simulink model "VAB_non_linear_Discrete"  (R2019b)
settings: Solver=FixedStepAuto  StartTime=0.0  StopTime=t_end  FixedStep=Ts  RelTol=1e-3
undefined symbols (not defined in the file or in its folder): Discrete, m_c_simulazione, phi_iniziale, phi_p_iniziale, phi_p_setpoint, phi_secondo, sensitivity_encoder, sensitivity_giroscopio, theta_iniziale, theta_p_iniziale, theta_secondo, Time, Ts
libraries: simulink x2, ctrlSharedLib x2
settings Model: Creator=miche  LastModifiedBy=AndreaCalegari

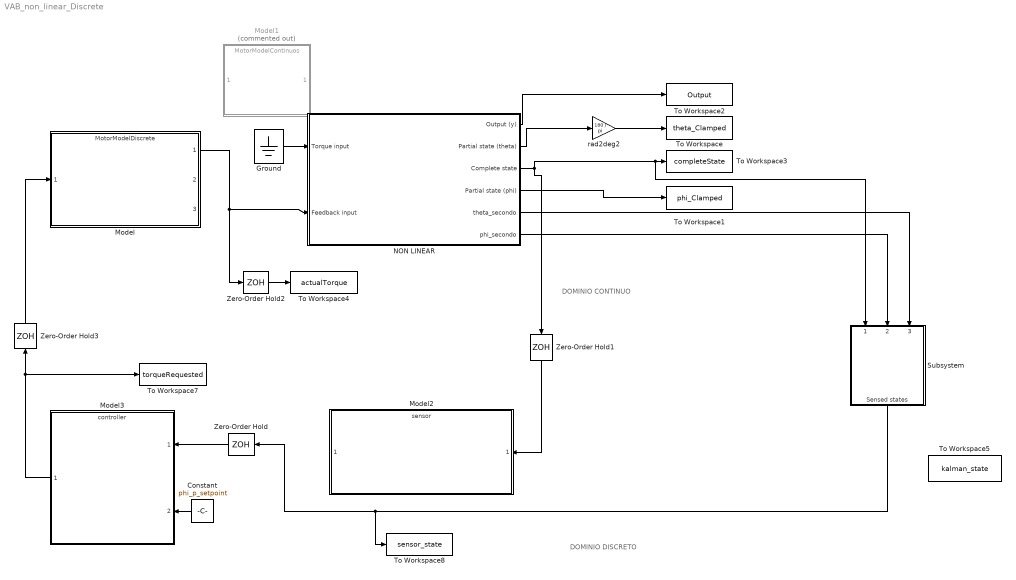
== system VAB_non_linear_Discrete ==
  note: DOMINIO DISCRETO
  note: DOMINIO CONTINUO
  Constant : Constant  Value=phi_p_setpoint
  Ground : Ground
  Model : ModelReference  ModelNameDialog=MotorModelDiscrete.slx  SimulationMode=Normal  ModelReferenceVersion=1.25
  Model1 : ModelReference  Commented=on  ModelNameDialog=MotorModelContinuos.slx  SimulationMode=Normal  ModelReferenceVersion=1.27
  Model2 : ModelReference  ModelNameDialog=sensor.slx  SimulationMode=Normal  ModelReferenceVersion=1.9
  Model3 : ModelReference  ModelNameDialog=controller.slx  SimulationMode=Normal  ModelReferenceVersion=1.24
  NON LINEAR : Subsystem
  Subsystem : Subsystem
  To Workspace : ToWorkspace  VariableName=theta_Clamped  SampleTime=-1
  To Workspace1 : ToWorkspace  VariableName=phi_Clamped  SampleTime=-1
  To Workspace2 : ToWorkspace  VariableName=Output  SampleTime=-1
  To Workspace3 : ToWorkspace  VariableName=completeState  SampleTime=-1
  To Workspace4 : ToWorkspace  VariableName=actualTorque  SampleTime=-1
  To Workspace5 : ToWorkspace  VariableName=kalman_state  SampleTime=-1
  To Workspace7 : ToWorkspace  VariableName=torqueRequested  SampleTime=-1
  To Workspace8 : ToWorkspace  VariableName=sensor_state  SampleTime=-1
  Zero-Order Hold{,1..3} (4 alike) : ZeroOrderHold  SampleTime=Ts
  rad2deg2 : Gain  Gain=180 / pi
  wires:
  Constant/1 -> Model3/2
  Zero-Order Hold1/1 -> Model2/1
  Model3/1 -> To Workspace7/1, Zero-Order Hold3/1
  NON LINEAR/1(Output (y)) -> To Workspace2/1
  Zero-Order Hold3/1 -> Model/1
  NON LINEAR/2(Partial state (theta)) -> rad2deg2/1
  rad2deg2/1 -> To Workspace/1
  NON LINEAR/4(Partial state (phi)) -> To Workspace1/1
  NON LINEAR/3("Complete state ") -> Zero-Order Hold1/1, Subsystem/1(Actual states), To Workspace3/1
  Model/1 -> Zero-Order Hold2/1, NON LINEAR/2(Feedback input)
  Ground/1 -> NON LINEAR/1(Torque input)
  Zero-Order Hold/1 -> Model3/1
  Zero-Order Hold2/1 -> To Workspace4/1
  NON LINEAR/6(phi_secondo) -> Subsystem/2(phi_secondo)
  NON LINEAR/5(theta_secondo) -> Subsystem/3("theta_sec ")
  Subsystem/1(Sensed states) -> To Workspace8/1, Zero-Order Hold/1

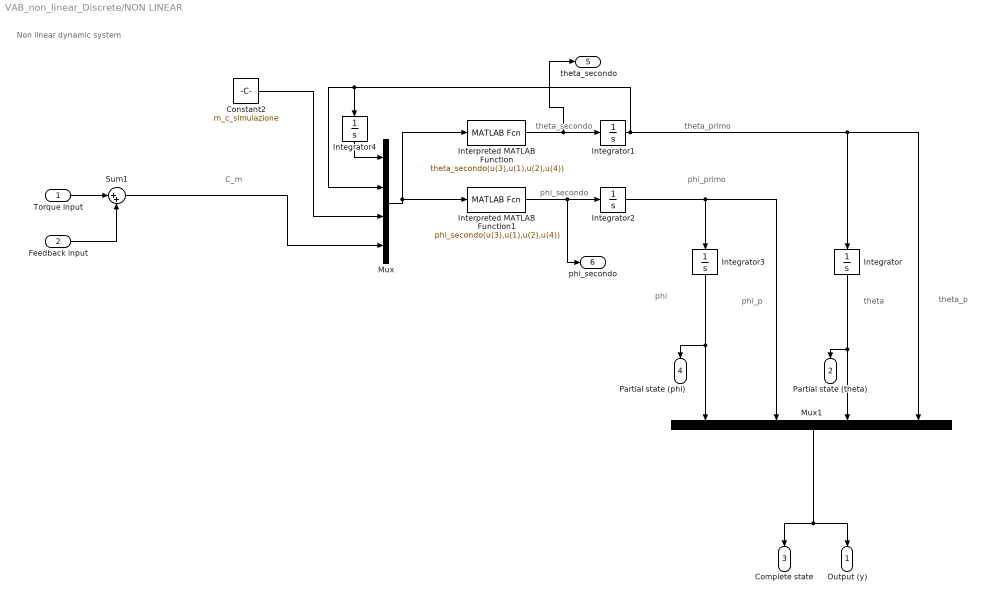
== system VAB_non_linear_Discrete/NON LINEAR ==
  note: Non linear dynamic system
  note: phi_primo
  note: phi
  note: theta_p
  note: theta
  note: phi_p
  note: phi_secondo
  note: C_m
  note: theta_secondo
  note: theta_primo
  Torque input : Inport  PortDimensions=1
  Feedback input : Inport  Port=2  PortDimensions=1
  Constant2 : Constant  Value=m_c_simulazione
  Integrator : Integrator  InitialCondition=theta_iniziale
  Integrator1 : Integrator  InitialCondition=theta_p_iniziale  UpperSaturationLimit=100  LowerSaturationLimit=-100
  Integrator2 : Integrator  InitialCondition=phi_p_iniziale
  Integrator3 : Integrator  InitialCondition=phi_iniziale
  Integrator4 : Integrator  InitialCondition=theta_iniziale
  Interpreted MATLAB Function : MATLABFcn  MATLABFcn=theta_secondo(u(3),u(1),u(2),u(4))  OutputDimensions=1
  Interpreted MATLAB Function1 : MATLABFcn  MATLABFcn=phi_secondo(u(3),u(1),u(2),u(4))  OutputDimensions=1
  Mux : Mux
      settings: DisplayOption=signals
  Mux1 : Mux
  Sum1 : Sum  Inputs=|++
  Output (y) : Outport
  Partial state (theta) : Outport  Port=2
  "Complete state " : Outport  Port=3
  Partial state (phi) : Outport  Port=4
  theta_secondo : Outport  Port=5
  phi_secondo : Outport  Port=6
  wires:
  Feedback input/1 -> Sum1/2
  Torque input/1 -> Sum1/1
  Integrator3/1 -> Partial state (phi)/1, Mux1/1
  Constant2/1 -> Mux/3
  Sum1/1 -> Mux/4
  Integrator4/1 -> Mux/1
  Interpreted MATLAB Function1/1 -> phi_secondo/1, Integrator2/1
  Integrator2/1 -> Mux1/2, Integrator3/1
  Integrator1/1 -> Integrator4/1, Mux/2, Mux1/4, Integrator/1
  Integrator/1 -> Partial state (theta)/1, Mux1/3
  Interpreted MATLAB Function/1 -> theta_secondo/1, Integrator1/1
  Mux1/1 -> Output (y)/1, "Complete state "/1
  Mux/1 -> Interpreted MATLAB Function/1, Interpreted MATLAB Function1/1

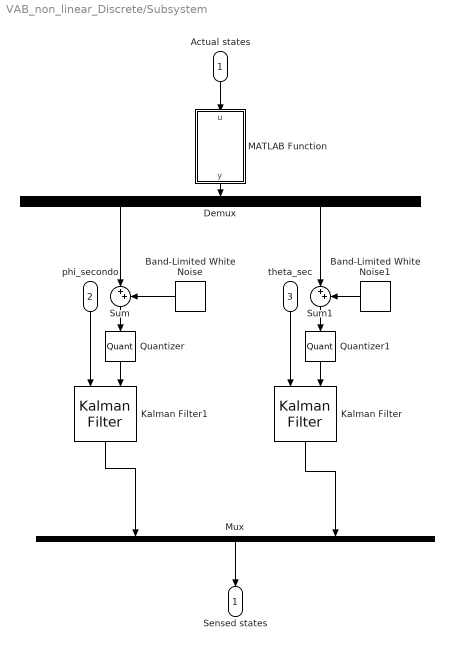
== system VAB_non_linear_Discrete/Subsystem ==
  Actual states : Inport  PortDimensions=4  SampleTime=Ts
  phi_secondo : Inport  Port=2  PortDimensions=1  SampleTime=Ts
  "theta_sec " : Inport  Port=3  PortDimensions=1  SampleTime=Ts
  Band-Limited White Noise : simulink/Sources/Band-Limited White Noise  Cov=[0.00000001]  Ts=0.001  seed=[23341]
  Band-Limited White Noise1 : simulink/Sources/Band-Limited White Noise  Cov=[0.00000001]  Ts=0.001  seed=[23341]
  Demux : Demux  Outputs=2
  Kalman Filter : ctrlSharedLib/Kalman Filter  TimeDomain=Discrete-Time  UseCurrentEstimator=on  ModelSource=Individual A, B, C, D matrices  ModelSourceVariable=ss(0.95,1,1,0,1)  A=[1,Ts;0,1]  B=[0.5*Ts*Ts;Ts]  C=[1,0]  D=0  NumberOfStates=1  NumberOfInputs=1  NumberOfOutputs=1  InitialEstimateSource=Dialog  X0=0  P0=10  UseK=off  UseGH=off  NumberOfProcessNoiseInputs=1  G=1  TimeInvariantG=on  H=0  TimeInvariantH=on  Q=0.0001  TimeInvariantQ=on  R=1  TimeInvariantR=on  N=0  TimeInvariantN=on  AddInputPort=on  AddEnablePort=off  OutputEstimatedY=off  OutputP=off  Ts=-1
      settings: SourceProductBaseCode=CT
  Kalman Filter1 : ctrlSharedLib/Kalman Filter  TimeDomain=Discrete-Time  UseCurrentEstimator=on  ModelSource=Individual A, B, C, D matrices  ModelSourceVariable=ss(0.95,1,1,0,1)  A=[1,Ts;0,1]  B=[0.5*Ts*Ts;Ts]  C=[1,0]  D=0  NumberOfStates=1  NumberOfInputs=1  NumberOfOutputs=1  InitialEstimateSource=Dialog  X0=0  P0=10  UseK=off  UseGH=off  NumberOfProcessNoiseInputs=1  G=1  TimeInvariantG=on  H=0  TimeInvariantH=on  Q=0.05  TimeInvariantQ=on  R=1  TimeInvariantR=on  N=0  TimeInvariantN=on  AddInputPort=on  AddEnablePort=off  OutputEstimatedY=off  OutputP=off  Ts=-1
      settings: SourceProductBaseCode=CT
  MATLAB Function : MATLAB Function  TreatAsAtomicUnit=on
  Mux : Mux  Inputs=2
  Quantizer : Quantizer  QuantizationInterval=1/sensitivity_encoder
  Quantizer1 : Quantizer  QuantizationInterval=1/sensitivity_giroscopio
  Sum : Sum  Inputs=|++
  Sum1 : Sum  Inputs=|++
  Sensed states : Outport
  wires:
  Actual states/1 -> MATLAB Function/1(u)
  MATLAB Function/1(y) -> Demux/1
  Kalman Filter1/1 -> Mux/1
  Sum/1 -> Quantizer/1
  phi_secondo/1 -> Kalman Filter1/1
  Band-Limited White Noise/1 -> Sum/2
  Demux/1 -> Sum/1
  Quantizer/1 -> Kalman Filter1/2
  "theta_sec "/1 -> Kalman Filter/1
  Kalman Filter/1 -> Mux/2
  Quantizer1/1 -> Kalman Filter/2
  Sum1/1 -> Quantizer1/1
  Demux/2 -> Sum1/1
  Band-Limited White Noise1/1 -> Sum1/2
  Mux/1 -> Sensed states/1

== matlab function VAB_non_linear_Discrete/Subsystem/MATLAB Function ==
  data: u input; y output
function y = fcn(u)

y = [u(1),u(3)];
